simulink model "CTC_CART_Tarea1"  (R2015a)
settings: Solver=ode45  StartTime=0.0  StopTime=3  RelTol=1e-3
values from neighbouring files (symbols this model uses):
  KP1 = 100000    [Inicio.m]
  KP2 = 85000    [Inicio.m]
  KP3 = 70000    [Inicio.m]
  KP4 = 70000    [Inicio.m]
  KV1 = 360    [Inicio.m]
  KV2 = 280    [Inicio.m]
  KV3 = 120    [Inicio.m]
  KV4 = 120    [Inicio.m]
  Ts = 0.001    [Inicio.m]    (also in circular.m)
undefined symbols (not defined in the file or in its folder): diferencia, MDI, mgd, mgi
libraries: simulink x1
settings Model: CovHtmlReporting=off  Creator=ANDRES Y MARCELA  LastModifiedBy=Shadow
settings DataIOCC: SignalLoggingSaveFormat=ModelDataLogs
settings OptimizationCC: ExpressionDepthLimit=2147483647
settings DebuggingCC: UnderspecifiedInitializationDetection=Classic  MergeDetectMultiDrivingBlocksExec=none  SolverPrmCheckMsg=warning  FcnCallInpInsideContextMsg=EnableAllAsWarning  StateNameClashWarn=warning
settings GRTTargetCC: CombineOutputUpdateFcns=off  GRTInterface=on

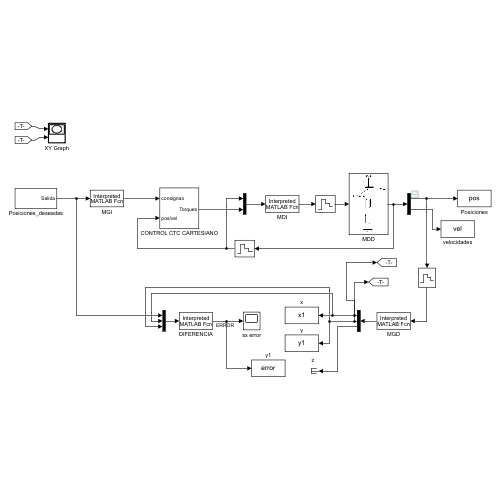
[thumbnail: Simulink's stored preview of the top-level diagram]
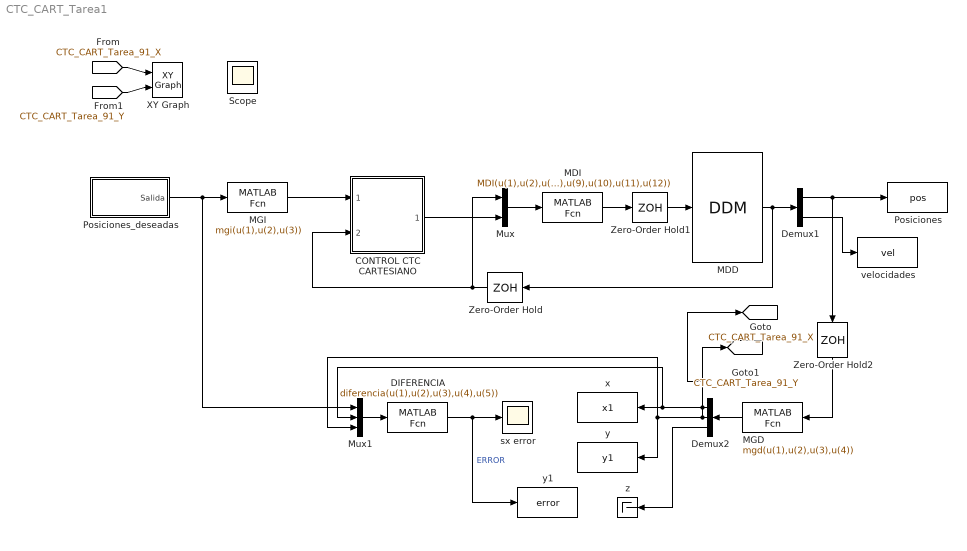
== system CTC_CART_Tarea1 ==
  CONTROL CTC CARTESIANO : Subsystem
  DIFERENCIA : MATLABFcn  MATLABFcn=diferencia(u(1),u(2),u(3),u(4),u(5))
  Demux1 : Demux  Outputs=2
  Demux2 : Demux  Outputs=3
  MDD : S-Function  FunctionName=DDM  Parameters=QI  SFunctionDeploymentMode=off  EnableBusSupport=off
      mask Display: image(imread('robot.jpg'))
  MDI : MATLABFcn  MATLABFcn=MDI(u(1),u(2),u(3),u(4),u(5),u(6),u(7),u(8),u(9),u(10),u(11),u(12))  OutputDimensions=4
  MGD : MATLABFcn  MATLABFcn=mgd(u(1),u(2),u(3),u(4))
  MGI : MATLABFcn  MATLABFcn=mgi(u(1),u(2),u(3))
  Mux : Mux  Inputs=2
  Mux1 : Mux  Inputs=3
  Posiciones : ToWorkspace  VariableName=pos  SampleTime=-1
  Posiciones_deseadas : Subsystem
  XY Graph : simulink/Sinks/XY Graph  xmin=-1  xmax=1  ymin=-1  ymax=1  st=-1
  Zero-Order Hold : ZeroOrderHold  SampleTime=Ts
  Zero-Order Hold1 : ZeroOrderHold  SampleTime=Ts
  Zero-Order Hold2 : ZeroOrderHold  SampleTime=Ts
  sx error : Scope
      settings: TimeRange=3  LimitDataPoints=on  MaxDataPoints=5000  SaveToWorkspace=off  SaveName=ScopeData  YMin=-0.00002  YMax=0.00021  SampleTime=-1
  velocidades : ToWorkspace  VariableName=vel  SampleTime=-1
  x : ToWorkspace  VariableName=x1  SampleTime=-1
  y : ToWorkspace  VariableName=y1  SampleTime=-1
  y1 : ToWorkspace  VariableName=error  SampleTime=-1
  z : Terminator
  Scope : Scope
      settings: TimeRange=auto  MaxDataPoints=5000  SaveToWorkspace=off  YMin=-1.02595  YMax=1.02595  SampleTime=-1
  tag scope: CTC_CART_Tarea_91_X=global, CTC_CART_Tarea_91_Y=global
  wires:
  MDD/1 -> Demux1/1, Zero-Order Hold/1
  Mux/1 -> MDI/1
  Zero-Order Hold/1 -> Mux/1, CONTROL CTC CARTESIANO/2(pos/vel)
  MDI/1 -> Zero-Order Hold1/1
  CONTROL CTC CARTESIANO/1(Torques) -> Mux/2
  MGI/1 -> CONTROL CTC CARTESIANO/1(consignas)
  Mux1/1 -> DIFERENCIA/1
  Demux1/1 -> Zero-Order Hold2/1, Posiciones/1
  MGD/1 -> Demux2/1
  Demux2/1 -> x/1, Mux1/2, [CTC_CART_Tarea_91_X]
  Demux2/2 -> y/1, Mux1/3, [CTC_CART_Tarea_91_Y]
  Demux2/3 -> z/1
  DIFERENCIA/1 -> sx error/1, y1/1  "ERROR"
  Zero-Order Hold2/1 -> MGD/1
  Demux1/2 -> velocidades/1
  Posiciones_deseadas/1(Salida) -> Mux1/1, MGI/1
  Zero-Order Hold1/1 -> MDD/1
  [CTC_CART_Tarea_91_X] -> XY Graph/1
  [CTC_CART_Tarea_91_Y] -> XY Graph/2

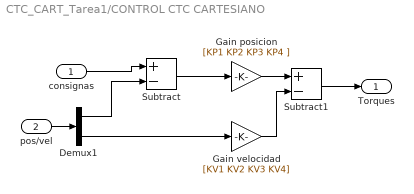
== system CTC_CART_Tarea1/CONTROL CTC CARTESIANO ==
  consignas : Inport
  pos/vel : Inport  Port=2
  Demux1 : Demux  Outputs=2
  Gain posicion : Gain  Gain=[KP1 KP2 KP3 KP4 ]
  Gain velocidad : Gain  Gain=[KV1 KV2 KV3 KV4]
  Subtract : Sum  Inputs=+-
  Subtract1 : Sum  Inputs=+-
  Torques : Outport
  wires:
  Subtract/1 -> Gain posicion/1
  Gain posicion/1 -> Subtract1/1
  Gain velocidad/1 -> Subtract1/2
  Demux1/1 -> Subtract/2
  Demux1/2 -> Gain velocidad/1
  consignas/1 -> Subtract/1
  pos/vel/1 -> Demux1/1
  Subtract1/1 -> Torques/1

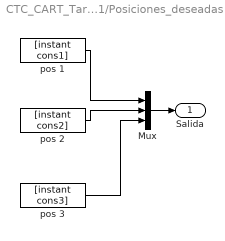
== system CTC_CART_Tarea1/Posiciones_deseadas ==
  Mux : Mux  Inputs=3
  pos 1 : FromWorkspace  VariableName=[instant cons1]  SampleTime=Ts  ZeroCross=off
  pos 2 : FromWorkspace  VariableName=[instant cons2]  SampleTime=Ts  ZeroCross=off
  pos 3 : FromWorkspace  VariableName=[instant cons3]  SampleTime=Ts  ZeroCross=off
  Salida : Outport
  wires:
  pos 1/1 -> Mux/1
  pos 2/1 -> Mux/2
  pos 3/1 -> Mux/3
  Mux/1 -> Salida/1
